simulink model "zad2"  (R2017b)
settings: Solver=VariableStepAuto  StartTime=0.0  StopTime=0  RelTol=1e-3
libraries: CPOiS_SourcesSinks x6, CPOiS_DataManipulation x2, CPOiS_General x1
settings Model: Creator=kstefanc  LastModifiedBy=kstefanc

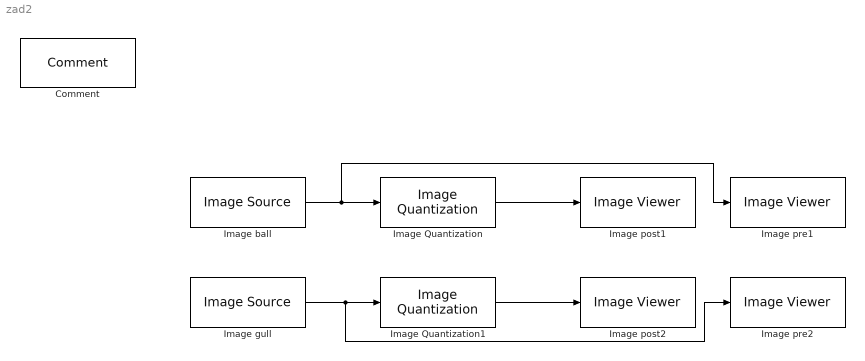
== system zad2 ==
  Comment : CPOiS_General/Comment
      settings: SourceProductName=CPOiS - Digital image and signal processing
  Image Quantization : CPOiS_DataManipulation/Image Quantization  LevelsNum=20
      settings: SourceProductName=CPOiS - Digital image and signal processing
  Image Quantization1 : CPOiS_DataManipulation/Image Quantization  LevelsNum=7
      settings: SourceProductName=CPOiS - Digital image and signal processing
  Image ball : CPOiS_SourcesSinks/Image Source  FileSelection=ball.png
      settings: SourceProductName=CPOiS - Digital image and signal processing
  "Image gull " : CPOiS_SourcesSinks/Image Source  FileSelection=gull.png
      settings: SourceProductName=CPOiS - Digital image and signal processing
  Image post1 : CPOiS_SourcesSinks/Image Viewer
      settings: SourceProductName=CPOiS - Digital image and signal processing
  Image post2 : CPOiS_SourcesSinks/Image Viewer
      settings: SourceProductName=CPOiS - Digital image and signal processing
  "Image pre1 " : CPOiS_SourcesSinks/Image Viewer
      settings: SourceProductName=CPOiS - Digital image and signal processing
  Image pre2 : CPOiS_SourcesSinks/Image Viewer
      settings: SourceProductName=CPOiS - Digital image and signal processing
  wires:
  Image Quantization/1 -> Image post1/1
  Image ball/1 -> Image Quantization/1, "Image pre1 "/1
  Image Quantization1/1 -> Image post2/1
  "Image gull "/1 -> Image Quantization1/1, Image pre2/1
